simulink model "hdl_model"  (R2024a)
settings: Solver=VariableStepAuto  StartTime=0.0  StopTime=SIM_TIME  RelTol=1e-3
undefined symbols (not defined in the file): BUFFER_LEN, SAMPLING_FREQ, signal_1
libraries: dspsrcs4 x1, hdlsllib x1, dsphdlxfrm2 x1, simulink_extras x1
settings Model: SimulationMode=accelerator  Creator=Jan Rosa  LastModifiedBy=Jan Rosa

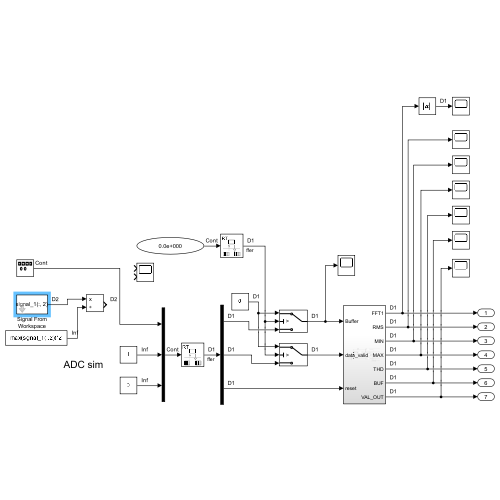
[thumbnail: Simulink's stored preview of the top-level diagram]
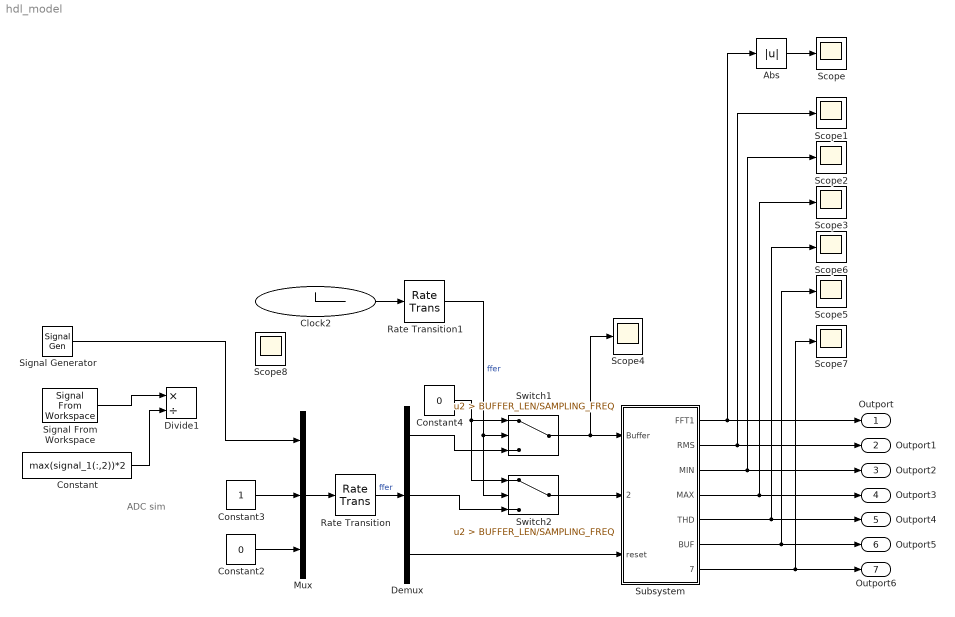
== system hdl_model ==
  note: ADC sim
  Abs : Abs  SaturateOnIntegerOverflow=off
  Clock2 : Clock
  Constant : Constant  Value=max(signal_1(:,2))*2
  Constant2 : Constant  Value=0
  Constant3 : Constant
  Constant4 : Constant  Value=0  SampleTime=1/SAMPLING_FREQ
  Demux : Demux  Outputs=3
  Divide1 : Product  Inputs=*/
  Mux : Mux  Inputs=3
  Rate Transition : RateTransition  Integrity=off  Deterministic=off  OutPortSampleTime=1/SAMPLING_FREQ
  Rate Transition1 : RateTransition  Integrity=off  Deterministic=off  OutPortSampleTime=1/SAMPLING_FREQ
  Scope{,1..7} (8 alike) : Scope
  Scope8 : Scope  NumInputPorts=2
  Signal Generator : SignalGenerator  WaveForm=square  Amplitude=1/2.001  Frequency=SAMPLING_FREQ/(16*16)
  Signal From Workspace : dspsrcs4/Signal From Workspace  X=signal_1(:, 2)  Ts=1.28/SAMPLING_FREQ  nsamps=1  OutputAfterFinalValue=Cyclic repetition  ignoreOrWarnInputAndFrameLengths=off  OutputFrames=off
  Subsystem : Subsystem
  Switch1 : Switch  Criteria=u2 > Threshold  Threshold=BUFFER_LEN/SAMPLING_FREQ  SaturateOnIntegerOverflow=off  InputSameDT=off
  Switch2 : Switch  Criteria=u2 > Threshold  Threshold=BUFFER_LEN/SAMPLING_FREQ  SaturateOnIntegerOverflow=off  InputSameDT=off
  Outport : Outport
  Outport1 : Outport  Port=2
  Outport2 : Outport  Port=3
  Outport3 : Outport  Port=4
  Outport4 : Outport  Port=5
  Outport5 : Outport  Port=6
  Outport6 : Outport  Port=7
  wires:
  Signal From Workspace/1 -> Divide1/1
  Constant/1 -> Divide1/2
  Constant3/1 -> Mux/2
  Constant2/1 -> Mux/3
  Subsystem/1(FFT1) -> Outport/1, Abs/1
  Subsystem/2(RMS) -> Outport1/1, Scope1/1
  Mux/1 -> Rate Transition/1
  Rate Transition/1 -> Demux/1  "ffer"
  Subsystem/3(MIN) -> Scope2/1, Outport2/1
  Subsystem/4(MAX) -> Scope3/1, Outport3/1
  Subsystem/5(THD) -> Scope6/1, Outport4/1
  Subsystem/7(VAL_OUT) -> Scope7/1, Outport6/1
  Abs/1 -> Scope/1
  Switch2/1 -> Subsystem/2(data_valid)
  Switch1/1 -> Scope4/1, Subsystem/1(Buffer)
  Demux/1 -> Switch1/3
  Demux/2 -> Switch2/3
  Clock2/1 -> Rate Transition1/1
  Constant4/1 -> Switch2/1, Switch1/1
  Demux/3 -> Subsystem/3(reset)
  Rate Transition1/1 -> Switch2/2, Switch1/2  "ffer"
  Subsystem/6(BUF) -> Outport5/1, Scope5/1
  Signal Generator/1 -> Mux/1

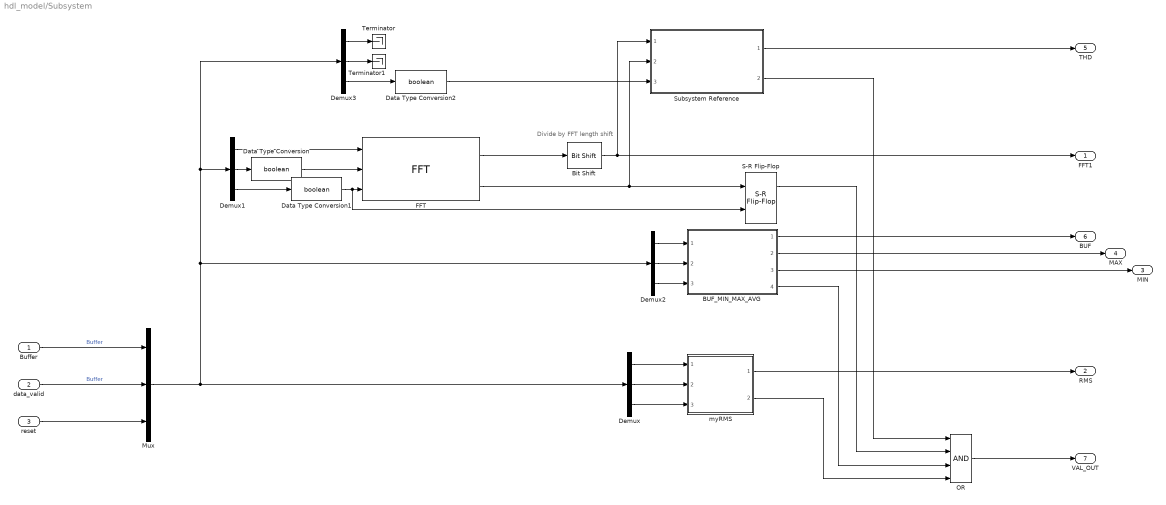
== system hdl_model/Subsystem ==
  note: Divide by FFT length shift
  Buffer : Inport
  data_valid : Inport  Port=2
  reset : Inport  Port=3
  BUF_MIN_MAX_AVG : Subsystem  ReferencedSubsystem=BUF_MIN_MAX_AVG
  Bit Shift : hdlsllib/Logic and Bit Operations/Bit Shift  mode=Shift Right Arithmetic  N=log2(BUFFER_LEN)
  Data Type Conversion : DataTypeConversion  OutDataTypeStr=boolean  SaturateOnIntegerOverflow=off  RndMeth=Floor
  Data Type Conversion1 : DataTypeConversion  OutDataTypeStr=boolean  SaturateOnIntegerOverflow=off  RndMeth=Floor
  Data Type Conversion2 : DataTypeConversion  OutDataTypeStr=boolean  SaturateOnIntegerOverflow=off  RndMeth=Floor
  Demux{,1..3} (4 alike) : Demux  Outputs=3
  FFT : dsphdlxfrm2/FFT  Architecture=Streaming Radix 2^2  FFTLengthSource=Property  FFTLength=BUFFER_LEN  FFTLengthMax=1024  ComplexMultiplication=Use 4 multipliers and 2 adders  BitReversedOutput=off  BitReversedInput=off  Normalize=off  SimulateUsing=Code generation  RoundingMethod=Floor  ResetInputPort=on  StartOutputPort=off  EndOutputPort=off
  Mux : Mux  Inputs=3
  OR : Logic  Inputs=4  IconShape=distinctive  AllPortsSameDT=off  OutDataTypeStr=boolean
  S-R Flip-Flop : simulink_extras/Flip Flops/S-R Flip-Flop  initial_condition=0
  Subsystem Reference : Subsystem  ReferencedSubsystem=myTHD
  Terminator : Terminator
  Terminator1 : Terminator
  myRMS : Subsystem  ReferencedSubsystem=myRMS
  FFT1 : Outport
  RMS : Outport  Port=2
  MIN : Outport  Port=3
  MAX : Outport  Port=4
  THD : Outport  Port=5
  BUF : Outport  Port=6
  VAL_OUT : Outport  Port=7
  wires:
  OR/1 -> VAL_OUT/1
  BUF_MIN_MAX_AVG/2 -> MAX/1
  BUF_MIN_MAX_AVG/3 -> MIN/1
  BUF_MIN_MAX_AVG/4 -> OR/3
  myRMS/1 -> RMS/1
  myRMS/2 -> OR/4
  Buffer/1 -> Mux/1  "Buffer"
  Demux/2 -> myRMS/2
  Demux/1 -> myRMS/1
  reset/1 -> Mux/3
  data_valid/1 -> Mux/2  "Buffer"
  Demux/3 -> myRMS/3
  Mux/1 -> Demux/1, Demux3/1, Demux1/1, Demux2/1
  Demux1/1 -> FFT/1
  Demux1/2 -> Data Type Conversion/1
  Demux1/3 -> Data Type Conversion1/1
  Demux2/1 -> BUF_MIN_MAX_AVG/1
  Demux2/2 -> BUF_MIN_MAX_AVG/2
  Demux2/3 -> BUF_MIN_MAX_AVG/3
  Demux3/3 -> Data Type Conversion2/1
  Demux3/1 -> Terminator/1
  Subsystem Reference/1 -> THD/1
  Subsystem Reference/2 -> OR/1
  Data Type Conversion1/1 -> S-R Flip-Flop/2, FFT/3
  Data Type Conversion/1 -> FFT/2
  FFT/1 -> Bit Shift/1
  Bit Shift/1 -> FFT1/1, Subsystem Reference/1
  FFT/2 -> S-R Flip-Flop/1, Subsystem Reference/2
  S-R Flip-Flop/1 -> OR/2
  Data Type Conversion2/1 -> Subsystem Reference/3
  Demux3/2 -> Terminator1/1
  BUF_MIN_MAX_AVG/1 -> BUF/1
